simulink model "ep4_4"  (R2023b)
settings: Solver=VariableStepAuto  StartTime=0.0  StopTime=100  RelTol=1e-3
settings Model: Creator=86186  LastModifiedBy=86186

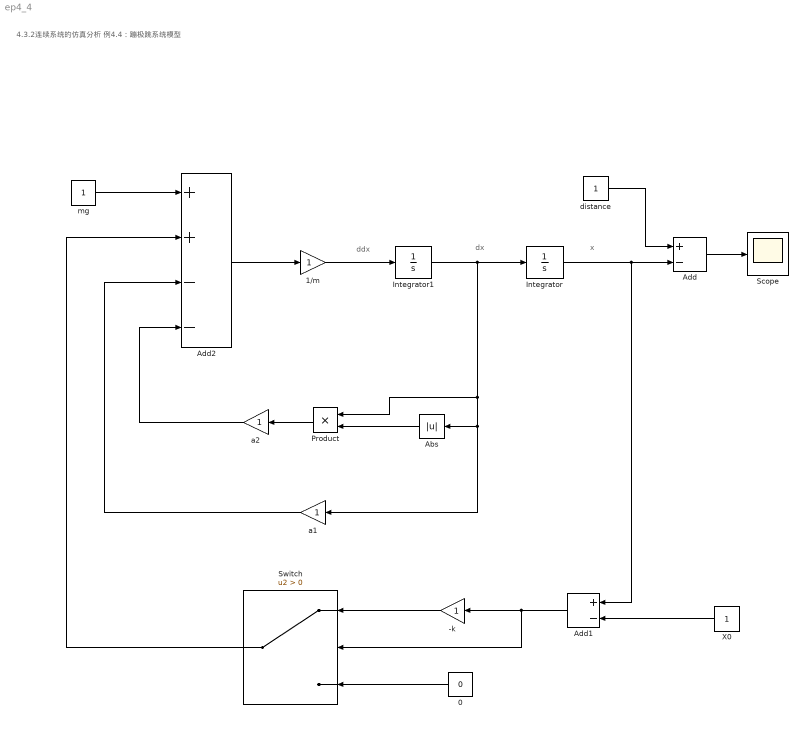
== system ep4_4 ==
  note: dx
  note: ddx
  note: 4.3.2连续系统的仿真分析
      | 例4.4：蹦极跳系统模型
  note: x
  -k : Gain
  0 : Constant  Value=0
  1/m : Gain
  Abs : Abs  SaturateOnIntegerOverflow=off
  Add : Sum  Inputs=+-
  Add1 : Sum  Inputs=+-
  Add2 : Sum  Inputs=++--
  Integrator : Integrator
  Integrator1 : Integrator
  Product : Product
  Scope : Scope
  Switch : Switch  Criteria=u2 > Threshold  SaturateOnIntegerOverflow=off  InputSameDT=off
  X0 : Constant
  a1 : Gain
  a2 : Gain
  distance : Constant
  mg : Constant
  wires:
  Add2/1 -> 1/m/1
  1/m/1 -> Integrator1/1
  Integrator1/1 -> Product/1, a1/1, Abs/1, Integrator/1
  Integrator/1 -> Add1/1, Add/2
  distance/1 -> Add/1
  Add/1 -> Scope/1
  Abs/1 -> Product/2
  Product/1 -> a2/1
  a2/1 -> Add2/4
  a1/1 -> Add2/3
  mg/1 -> Add2/1
  Switch/1 -> Add2/2
  -k/1 -> Switch/1
  Add1/1 -> Switch/2, -k/1
  0/1 -> Switch/3
  X0/1 -> Add1/2
